simulink model "angle_speed_to_pwm"  (R2017a)
settings: Solver=VariableStepAuto  StartTime=0.0  StopTime=50000  RelTol=1e-3
libraries: hdlsllib x4, simulink x1
settings Model: Creator=Ryan Corkery  LastModifiedBy=Ryan Corkery

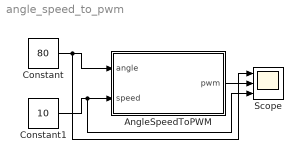
== system angle_speed_to_pwm ==
  AngleSpeedToPWM : Subsystem
  Constant : Constant  Value=80  OutDataTypeStr=uint8  SampleTime=1
  Constant1 : Constant  Value=10  OutDataTypeStr=uint8  SampleTime=1
  Scope : Scope  NumInputPorts=3
  wires:
  Constant/1 -> Scope/2, AngleSpeedToPWM/1(angle)
  Constant1/1 -> Scope/3, AngleSpeedToPWM/2("speed ")
  AngleSpeedToPWM/1(pwm) -> Scope/1

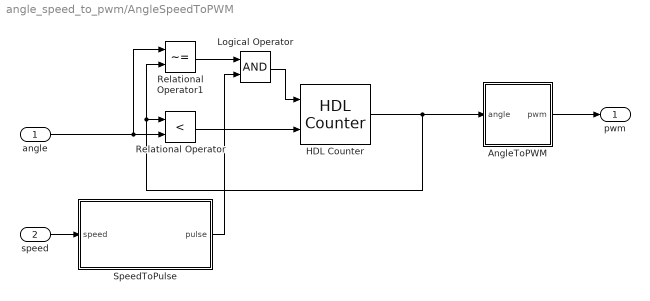
== system angle_speed_to_pwm/AngleSpeedToPWM ==
  angle : Inport  OutDataTypeStr=uint8
  "speed " : Inport  Port=2  OutDataTypeStr=uint8
  AngleToPWM : Subsystem
  HDL Counter : hdlsllib/HDL Operations/HDL Counter  CountType=Count limited  CountInit=90  CountStep=1  CountMax=180  CountFromType=Specify  CountFrom=0  CountResetPort=off  CountLoadPort=off  CountEnbPort=on  CountDirPort=on  CountDataType=Unsigned  CountWordLen=8  CountFracLen=0  CountSampTime=1
      settings: SourceProductName=HDL Coder  SourceProductBaseCode=HD
  Logical Operator : Logic  AllPortsSameDT=off  OutDataTypeStr=boolean
  Relational Operator : RelationalOperator  Operator=<  OutDataTypeStr=boolean  RndMeth=Simplest
  Relational Operator1 : RelationalOperator  Operator=~=  OutDataTypeStr=boolean  RndMeth=Simplest
  SpeedToPulse : Subsystem
  pwm : Outport  OutDataTypeStr=boolean
  wires:
  Relational Operator1/1 -> Logical Operator/1
  AngleToPWM/1(pwm) -> pwm/1
  HDL Counter/1 -> AngleToPWM/1("angle "), Relational Operator1/2, Relational Operator/1
  SpeedToPulse/1(pulse) -> Logical Operator/2
  Relational Operator/1 -> HDL Counter/2
  angle/1 -> Relational Operator1/1, Relational Operator/2
  Logical Operator/1 -> HDL Counter/1
  "speed "/1 -> SpeedToPulse/1(speed)

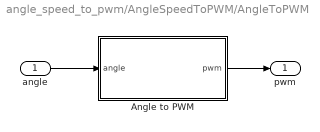
== system angle_speed_to_pwm/AngleSpeedToPWM/AngleToPWM ==
  "angle " : Inport  OutDataTypeStr=uint8
  Angle to PWM : Subsystem
  pwm : Outport
  wires:
  "angle "/1 -> Angle to PWM/1("angle ")
  Angle to PWM/1(pwm) -> pwm/1

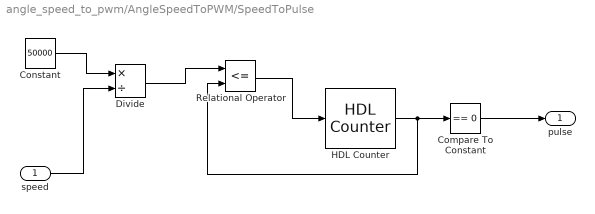
== system angle_speed_to_pwm/AngleSpeedToPWM/SpeedToPulse ==
  speed : Inport  OutDataTypeStr=uint8
  Compare To Constant : simulink/Logic and Bit Operations/Compare To Constant  relop===  const=0  OutDataTypeStr=boolean
  Constant : Constant  Value=50000  OutDataTypeStr=uint32  SampleTime=1
  Divide : Product  Inputs=*/  SaturateOnIntegerOverflow=on  RndMeth=Zero
  HDL Counter : hdlsllib/HDL Operations/HDL Counter  CountType=Free running  CountInit=0  CountStep=1  CountMax=25  CountFromType=Initial value  CountFrom=0  CountResetPort=on  CountLoadPort=off  CountEnbPort=off  CountDirPort=off  CountDataType=Unsigned  CountWordLen=32  CountFracLen=0  CountSampTime=1
      settings: SourceProductName=HDL Coder  SourceProductBaseCode=HD
  Relational Operator : RelationalOperator  Operator=<=  OutDataTypeStr=boolean  RndMeth=Nearest
  pulse : Outport
  wires:
  Divide/1 -> Relational Operator/1
  Compare To Constant/1 -> pulse/1
  HDL Counter/1 -> Relational Operator/2, Compare To Constant/1
  Relational Operator/1 -> HDL Counter/1
  Constant/1 -> Divide/1
  speed/1 -> Divide/2

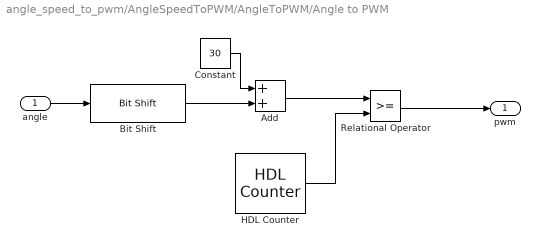
== system angle_speed_to_pwm/AngleSpeedToPWM/AngleToPWM/Angle to PWM ==
  "angle " : Inport  OutDataTypeStr=uint8
  Add : Sum
  Bit Shift : hdlsllib/HDL Operations/Bit Shift  mode=Shift Right Logical  N=1
      settings: SourceProductName=HDL Coder  SourceProductBaseCode=HD
  Constant : Constant  Value=30  OutDataTypeStr=uint8
  HDL Counter : hdlsllib/HDL Operations/HDL Counter  CountType=Count limited  CountInit=0  CountStep=1  CountMax=1000  CountFromType=Initial value  CountFrom=0  CountResetPort=off  CountLoadPort=off  CountEnbPort=off  CountDirPort=off  CountDataType=Unsigned  CountWordLen=16  CountFracLen=0  CountSampTime=1
      settings: SourceProductName=HDL Coder  SourceProductBaseCode=HD
  Relational Operator : RelationalOperator  OutDataTypeStr=boolean  RndMeth=Simplest
  pwm : Outport
  wires:
  HDL Counter/1 -> Relational Operator/2
  Relational Operator/1 -> pwm/1
  Add/1 -> Relational Operator/1
  Bit Shift/1 -> Add/2
  Constant/1 -> Add/1
  "angle "/1 -> Bit Shift/1
